simulink model "dsppitchtime_win32"  (Simulink 6.0)
settings: Solver=FixedStepDiscrete  StartTime=0.0  StopTime=4  RelTol=1e-3
libraries: dspsigops x5, dspmtrx3 x4, dspobslib x4, dspwin32 x2, dspxfrm3 x2, dspsigattribs x1, simulink x1, dspbuff3 x1, dspsrcs4 x1, dspswit3 x1
settings Model: Creator=mkhan  LastModifiedBy=mkhan  ExtModeAutoUpdateStatusClock=off  ProdHWDeviceType=Specified
settings DataIOCC: LimitDataPoints=off  SaveTime=off  OutputSaveName=y_pnt  SignalLoggingName=logsOut
settings OptimizationCC: InlineParams=on
settings DebuggingCC: CheckExecutionContextPreStartOutputMsg=on  CheckExecutionContextRuntimeOutputMsg=on  SolverPrmCheckMsg=none
settings HardwareCC: ProdHWDeviceType=Specified
settings SFSimCC: SFSimApplyToAllLibs=on  SFSimBuildMode=Incremental

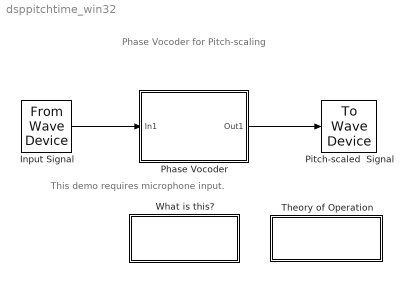
== system dsppitchtime_win32 ==
  note: Phase Vocoder for Pitch-scaling
  note: This demo requires microphone input.
  Input Signal : dspwin32/From Wave Device  SampleRate=8000  UserRate=16000  SampleWidth=16  Stereo=off  SamplesPerFrame=64  QueueDuration=3  useDefaultDevice=on  userDeviceID=INPUTDEVS  dType=double
  Phase Vocoder : Subsystem  PropExecContextAcrossSSBoundary=on  mask(Phase Vocoder){ana_hopSize=64, winLen=256, syn_hopSize=90}
      mask prompts: ana_hopSize "Analysis hop-size (i.e., temporal shift of analysis window) (in samples):"; winLen "Window size (in samples):"; syn_hopSize "Synthesis hop-size (i.e., temporal shift of synthesis window) (in samples):"
      mask help:
      | Algorithm for time-stretching and pitch-scaling of an audio signal. Time-stretching changes the speed of an audio signal without affecting its pitch. Pitch-scaling changes the pitch of an audio signal without affecting its speed.
      |
      | The pitch-scaling and time-stretching factors are defined by the ratio of the Synthesis hop-size parameter to the Analysis hop-size parameter.
      |
      | The Window size parameter must meet the following two requirements:
      | - log2(Window size) must be a positive integer
      | - Window size must be greater than both the Analysis hop-size and the Synthesis hop-size parameter values.
      mask Display: disp('Phase Vocoder')
  Pitch-scaled  Signal : dspwin32/To Wave Device  bufDuration=2  initDelay=0.1  useDefaultDevice=on  userDeviceID=OUTPUTDEVS  enable24Bit=off
  Theory of Operation : Subsystem  PropExecContextAcrossSSBoundary=on
      mask Type: Theory of Operation
      mask Display: disp('Theory of\nOperation')
  What is this? : Subsystem  PropExecContextAcrossSSBoundary=on
      mask Type: Frame-Based Simulation Info
      mask Display: disp('What is this?')
  wires:
  Phase Vocoder/1(Out1) -> Pitch-scaled  Signal/1
  Input Signal/1 -> Phase Vocoder/1(In1)

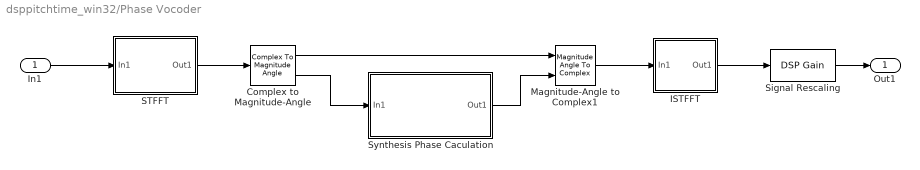
== system dsppitchtime_win32/Phase Vocoder ==
  In1 : Inport  LatchInput=off
  Complex to Magnitude-Angle : ComplexToMagnitudeAngle
  ISTFFT : Subsystem  PropExecContextAcrossSSBoundary=on
      mask Display: disp('Overlap\nIST-FFT')
  Magnitude-Angle to Complex1 : MagnitudeAngleToComplex
  STFFT : Subsystem  PropExecContextAcrossSSBoundary=on
      mask Display: disp('Overlap\nST-FFT')
  Signal Rescaling : dspobslib/DSP Gain  gainValue=1/(winLen*sum(hanning(winLen,'periodic').^2)/syn_hopSize)  roundingMode=Floor  overflowMode=off
  Synthesis Phase Caculation : Subsystem  PropExecContextAcrossSSBoundary=on  mask{ana_hopSize=ana_hopSize, syn_hopSize=syn_hopSize, winLen=winLen}
      mask prompts: ana_hopSize "Analysis hop size:"; syn_hopSize "Synthesis hop size:"; winLen "Window size:"
      mask Display: disp('Synthesis\nPhase\nCalculation')
  Out1 : Outport
  wires:
  In1/1 -> STFFT/1(In1)
  STFFT/1(Out1) -> Complex to Magnitude-Angle/1
  Magnitude-Angle to Complex1/1 -> ISTFFT/1(In1)
  ISTFFT/1(Out1) -> Signal Rescaling/1
  Complex to Magnitude-Angle/2 -> Synthesis Phase Caculation/1(In1)
  Complex to Magnitude-Angle/1 -> Magnitude-Angle to Complex1/1
  Synthesis Phase Caculation/1(Out1) -> Magnitude-Angle to Complex1/2
  Signal Rescaling/1 -> Out1/1

== system dsppitchtime_win32/Theory of Operation ==
  note: This simulation demonstrates the pitch-scaling effect applied to audio
      | signal using Phase Vocoder. To see the implementation "Look Under"
      | the "Phase Vocoder" block by selecting the block and either hitting
      | "ctrl+u", or right clicking on the block and selecting "Look Under Mask."
      |
      | For further information you may also refer to the following paper:
      | A. D. Gotzen, N. Bernardini and D. Arfib, "Traditional Implementations
      | of a Phase-Vocoder: The Tricks of the Trade," Proc. of the COST G-6
      | Conference on Digital Audio Effects (DAFX-00), Verona, Italy,
      | December 7-9, 2000.

== system dsppitchtime_win32/What is this? ==
  note: This simulation demonstrates how to use a phase vocoder
      | to implement real-time pitch-scaling of an audio signal.
      | This model can only be run on WIN32 platforms.
      |
      | This demo requires microphone input. The model modifies the
      | pitch of the input signal and outputs it to a Windows audio
      | device while the simulation is running.
      |
      | Double-click the Phase Vocoder block. Change the Synthesis
      | hop-size parameter to 64, the same value as the Analysis hop-size
      | parameter. Run the simulation and listen to the Pitch-scaled Signal.
      |
      | Double-click the Phase Vocoder block. Change the Synthesis
      | hop-size parameter to 48. Run the simulation and listen to the
      | Pitch-scaled Signal.

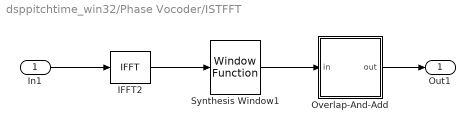
== system dsppitchtime_win32/Phase Vocoder/ISTFFT ==
  In1 : Inport  LatchInput=off
  IFFT2 : dspxfrm3/IFFT  DialogController=dspDDGCreate  DialogControllerArgs=DataTag0  CompMethod=Table lookup  TableOpt=Speed  BitRevOrder=off  cs_in=on  SkipNorm=on  mode=Complex  firstCoeffMode=User-defined  firstCoeffWordLength=16  firstCoeffFracLength=15  roundingMode=Floor  overflowMode=off
  Overlap-And-Add : Subsystem  PropExecContextAcrossSSBoundary=on  mask(Overlap-And-Add){L=syn_hopSize}
      mask prompts: L "Number of new points in each frame"
      mask help: Performs overlap-and-add on the input signal. Disjoint frames of the input signal are overlapped with each other for a specified number of points and summed.
      mask Display: disp('Overlap\nAnd\nAdd')
  Synthesis Window1 : dspsigops/Window Function  DialogController=dspDDGCreate  DialogControllerArgs=DataTag1  winmode=Apply window to input  wintype=Hanning  sampmode=Continuous  samptime=1  N=64  Rs=50  beta=10  winsamp=Periodic  UserWindow=hamming  OptParams=off  UserParams={1.0}  dataType=double  isSigned=on  wordLen=16  udDataType=sfix(16)  fracBitsMode=Best precision  numFracBits=15  roundingMode=Floor  overflowMode=off
  Out1 : Outport
  wires:
  IFFT2/1 -> Synthesis Window1/1
  Overlap-And-Add/1(out) -> Out1/1
  In1/1 -> IFFT2/1
  Synthesis Window1/1 -> Overlap-And-Add/1(in)

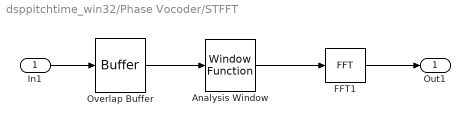
== system dsppitchtime_win32/Phase Vocoder/STFFT ==
  In1 : Inport  LatchInput=off
  Analysis Window : dspsigops/Window Function  winmode=Apply window to input  wintype=Hanning  sampmode=Continuous  samptime=1  N=64  Rs=50  beta=10  winsamp=Periodic  UserWindow=hamming  OptParams=off  UserParams={1.0}  dataType=double  wordLen=16  udDataType=sfix(16)  fracBitsMode=Best precision  numFracBits=15  roundingMode=Floor  overflowMode=off
  FFT1 : dspxfrm3/FFT  CompMethod=Table lookup  TableOpt=Speed  BitRevOrder=off  SkipNorm=off  firstCoeffMode=User-defined  firstCoeffWordLength=16  firstCoeffFracLength=15  roundingMode=Floor  overflowMode=off
  Overlap Buffer : dspbuff3/Buffer  N=winLen  V=winLen-ana_hopSize  ic=0
  Out1 : Outport
  wires:
  Overlap Buffer/1 -> Analysis Window/1
  FFT1/1 -> Out1/1
  In1/1 -> Overlap Buffer/1
  Analysis Window/1 -> FFT1/1

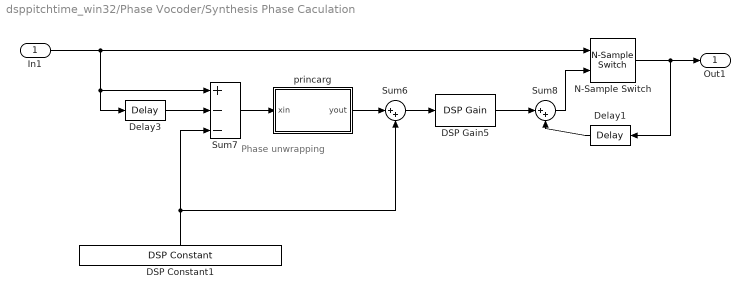
== system dsppitchtime_win32/Phase Vocoder/Synthesis Phase Caculation ==
  note: Phase unwrapping
  In1 : Inport  LatchInput=off
  DSP Constant1 : dspsrcs4/DSP Constant  Orientation=up  Value=2*pi*ana_hopSize*[0:winLen-1]'/winLen  SampleMode=Discrete  discreteOutput=Sample-based  continuousOutput=Sample-based  sampTime=64/8000  framePeriod=2  dataType=Inherit from 'Constant value'  isSigned=on  wordLen=16  udDataType=sfix(16)  fracBitsMode=Best precision  numFracBits=15  InterpretAs1D=-inf  Ts=-inf  FramebasedOutput=-inf
  DSP Gain5 : dspobslib/DSP Gain  gainValue=syn_hopSize/ana_hopSize  roundingMode=Floor  overflowMode=off
  Delay1 : dspsigops/Delay  Orientation=left  dly_unit=Frames  delay=1  ic_detail=on  dif_ic_for_ch=off  dif_ic_for_dly=off  ic=0  reset_popup=None
  Delay3 : dspsigops/Delay  dly_unit=Frames  delay=1  ic_detail=on  dif_ic_for_ch=off  dif_ic_for_dly=off  ic=0  reset_popup=None
  N-Sample Switch : dspswit3/N-Sample Switch  N=1  reset=off  TriggerType=Rising edge  Ts=-1
  Sum6 : Sum  Inputs=|++  SaturateOnIntegerOverflow=on
  Sum7 : Sum  Inputs=+--  SaturateOnIntegerOverflow=on
  Sum8 : Sum  Inputs=|++  SaturateOnIntegerOverflow=on
  princarg : Subsystem  PropExecContextAcrossSSBoundary=on
      mask Display: disp('Principal\nArgument');
  Out1 : Outport
  wires:
  In1/1 -> N-Sample Switch/1, Delay3/1, Sum7/1
  Delay3/1 -> Sum7/2
  DSP Constant1/1 -> Sum7/3, Sum6/2
  Sum7/1 -> princarg/1(xin)
  princarg/1(yout) -> Sum6/1
  Sum6/1 -> DSP Gain5/1
  DSP Gain5/1 -> Sum8/1
  N-Sample Switch/1 -> Delay1/1, Out1/1
  Delay1/1 -> Sum8/2
  Sum8/1 -> N-Sample Switch/2

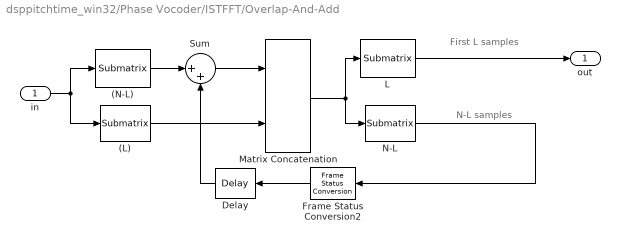
== system dsppitchtime_win32/Phase Vocoder/ISTFFT/Overlap-And-Add ==
  note: First L samples
  note: N-L samples
  in : Inport  LatchInput=off
  (L) : dspmtrx3/Submatrix  RowSpan=Range of rows  RowStartMode=Offset from last  RowStartIndex=L-1  RowEndMode=Last  RowEndIndex=1  ColSpan=All columns  ColStartMode=First  ColStartIndex=1  ColEndMode=Last  ColEndIndex=1
  (N-L) : dspmtrx3/Submatrix  RowSpan=Range of rows  RowStartMode=First  RowStartIndex=1  RowEndMode=Offset from last  RowEndIndex=L  ColSpan=All columns  ColStartMode=First  ColStartIndex=1  ColEndMode=Last  ColEndIndex=1
  Delay : dspsigops/Delay  Orientation=left  dly_unit=Samples  delay=1  ic_detail=off  dif_ic_for_ch=off  dif_ic_for_dly=off  ic=0  reset_popup=None
  Frame Status Conversion2 : dspsigattribs/Frame Status Conversion  Orientation=left  growRefPort=off  outframe=Sample-based
  L : dspmtrx3/Submatrix  RowSpan=Range of rows  RowStartMode=First  RowStartIndex=1  RowEndMode=Index  RowEndIndex=L  ColSpan=All columns  ColStartMode=First  ColStartIndex=1  ColEndMode=Last  ColEndIndex=1
  Matrix Concatenation : simulink/Math Operations/Matrix Concatenation  numInports=2  catMethod=Vertical
  N-L : dspmtrx3/Submatrix  RowSpan=Range of rows  RowStartMode=Index  RowStartIndex=L+1  RowEndMode=Last  RowEndIndex=1  ColSpan=All columns  ColStartMode=First  ColStartIndex=1  ColEndMode=Last  ColEndIndex=1
  Sum : Sum  Inputs=|++  SaturateOnIntegerOverflow=on  InputSameDT=on
  out : Outport
  wires:
  L/1 -> out/1
  Sum/1 -> Matrix Concatenation/1
  (N-L)/1 -> Sum/1
  Delay/1 -> Sum/2
  (L)/1 -> Matrix Concatenation/2
  N-L/1 -> Frame Status Conversion2/1
  Matrix Concatenation/1 -> L/1, N-L/1
  in/1 -> (L)/1, (N-L)/1
  Frame Status Conversion2/1 -> Delay/1

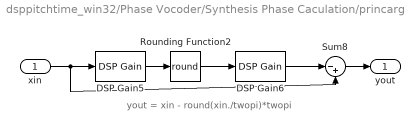
== system dsppitchtime_win32/Phase Vocoder/Synthesis Phase Caculation/princarg ==
  note: yout = xin - round(xin./twopi)*twopi
  xin : Inport  LatchInput=off
  DSP Gain5 : dspobslib/DSP Gain  gainValue=1/(2*pi)  roundingMode=Floor  overflowMode=off
  DSP Gain6 : dspobslib/DSP Gain  gainValue=2*pi  roundingMode=Floor  overflowMode=off
  Rounding Function2 : Rounding  Operator=round
  Sum8 : Sum  Inputs=|-+  SaturateOnIntegerOverflow=on
  yout : Outport
  wires:
  xin/1 -> Sum8/2, DSP Gain5/1
  DSP Gain5/1 -> Rounding Function2/1
  Rounding Function2/1 -> DSP Gain6/1
  DSP Gain6/1 -> Sum8/1
  Sum8/1 -> yout/1
